simulink model "I_HeatConductionThroughInsulatedIronRod"  (R2024b)
settings: Solver=VariableStepAuto  StartTime=0.0  StopTime=5  MaxStep=100  RelTol=1e-3  AbsTol=1e-3  EnableMultiTasking=on
PreLoadFcn:
  | if ~exist('T_base', 'var')   T_base= 100;   end % [degC]
  | if ~exist('L', 'var')        L= 0.2;        end % [m]
  | if ~exist('D', 'var')        D= 0.025;      end % [m]
  | if ~exist('A', 'var')        A= pi*D^2/4;   end % [m^2]
  | if ~exist('k', 'var')        k= 80.2;       end % [W/(K*m)]
  | if ~exist('Q_case_1', 'var') Q_case_1= 18;  end % [W]
libraries: fl_lib x6, nesl_utility x2
Description:
  | Steady State Heat Conduction Through Insulated Iron Rod
settings Model: Creator=The MathWorks, Inc.  LastModifiedBy=mvahab
settings SolverCC: AutoScaleAbsTol=off  AlgebraicLoopSolver=TrustRegion
settings DataIOCC: LimitDataPoints=on  SaveFormat=Array  ReturnWorkspaceOutputs=off
settings OptimizationCC: LifeSpan=inf
settings DebuggingCC: SolverPrmCheckMsg=warning  UnconnectedInputMsg=warning  UnconnectedOutputMsg=warning  UnconnectedLineMsg=warning  AllowSymbolicDim=off  PregeneratedLibrarySubsystemCodeDiagnostic=none  SFUnexpectedBacktrackingDiag=warning  SFNoUnconditionalDefaultTransitionDiag=warning  SFExecutionAtInitializationDiag=none  ArithmeticOperatorsInVariantConditions=warning
settings HardwareCC: ProdBitPerPointer=32  ProdBitPerSizeT=32  ProdBitPerPtrDiffT=32  ProdLargestAtomicFloat=None  ProdIntDivRoundTo=Undefined  ProdEndianess=Unspecified  ProdWordSize=32  ProdHWDeviceType=32-bit Generic
settings ModelReferenceCC: EnableRefExpFcnMdlSchedulingChecks=on  PropagateSignalLabelsOutOfModel=off
settings SFSimCC: SimUseLocalCustomCode=off  CustomCodeUndefinedFunction=UseInterfaceOnly
settings RTWCC: RTWUseLocalCustomCode=off  GPUComputeCapability=3.5  DLArmComputeVersion=19.05
settings CodeAppCC: StateflowObjectComments=on
settings GRTTargetCC: TargetLangStandard=C89/C90 (ANSI)
settings ConfigComp: CovMetricSettings=dw  CovSaveCumulativeToWorkspaceVar=on  CovSaveSingleToWorkspaceVar=on  CovExternalEMLEnable=off  CovSFcnEnable=off
settings SimscapeCC: SimscapeLogType=all  SimscapeLogSimulationStatistics=on  SimscapeLogName=simlog_HeatConductionThroughInsulatedIronRod  SimscapeLogDataHistory=10000

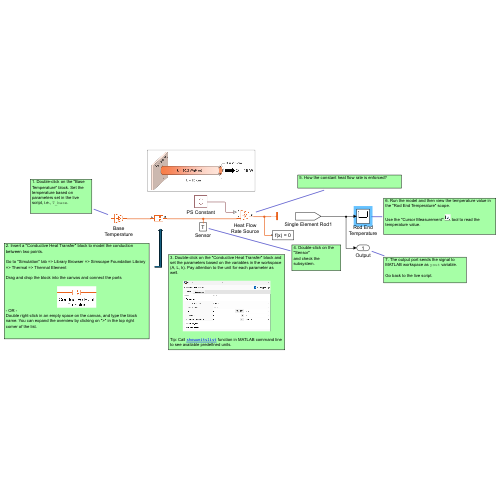
[thumbnail: Simulink's stored preview of the top-level diagram]
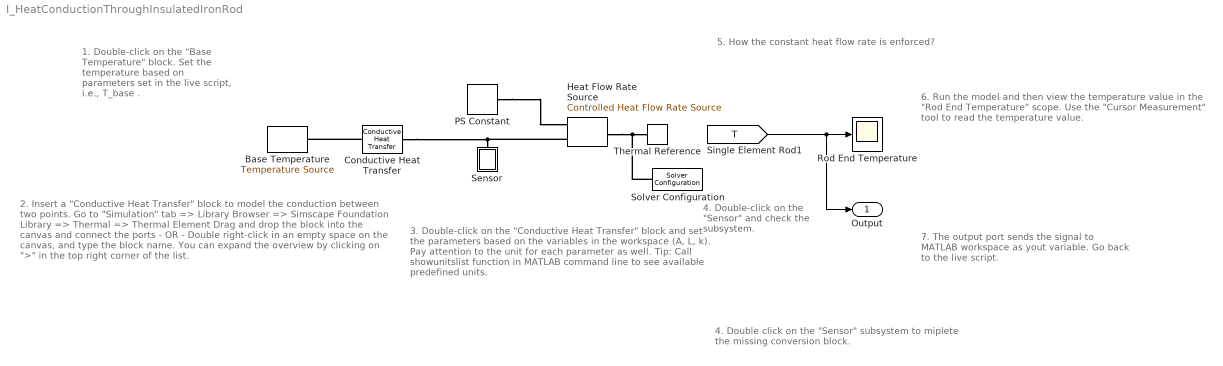
== system I_HeatConductionThroughInsulatedIronRod ==
  note: 2. Insert a "Conductive Heat Transfer" block to model the conduction between two points.
      |
      | Go to "Simulation" tab => Library Browser => Simscape Foundation Library => Thermal => Thermal Element
      |
      | Drag and drop the block into the canvas and connect the ports
      |
      | - OR -
      | Double right-click in an empty space on the canvas, and type the block name. You can expand the overview by clicking on ">" in the top right corner of the list.
  note: 3. Double-click on the "Conductive Heat Transfer" block and set the parameters based on the variables in the workspace (A, L, k). Pay attention to the unit for each parameter as well.
      |
      | Tip: Call showunitslist function in MATLAB command line to see available predefined units.
  note: 4. Double-click on the "Sensor"
      | and check the subsystem.
  note: 1. Double-click on the "Base Temperature" block. Set the temperature based on parameters set in the live script, i.e., T_base .
  note: 4. Double click on the "Sensor" subsystem to miplete the missing conversion block.
  note: 6. Run the model and then view the temperature value in the "Rod End Temperature" scope.
      |
      | Use the "Cursor Measurement" tool to read the temperature value.
  note: 7. The output port sends the signal to MATLAB workspace as yout variable.
      |
      | Go back to the live script.
  note: 5. How the constant heat flow rate is enforced?
  Base Temperature : fl_lib/Thermal/Thermal Sources/Temperature Source  temperature=T_base degC
  Conductive Heat Transfer : fl_lib/Thermal/Thermal Elements/Conductive Heat Transfer  thermal_type=foundation.enum.ConstantVariableTabulated.Constant  wall_geometry=foundation.enum.ConductionWallGeometry.Planar  area=A m^2  thickness=L m  d_in=0.05 m  d_out=0.1 m  L=1 m  th_cond_min=10 W/(K*m)  th_cond=k W/(K*m)  th_cond_TLU=[413, 401, 392, 383, 371, 357, 342] W/(K*m)  temp_TLU=[200, 273, 400, 600, 800, 1000, 1200] K  T_specify=off  T_priority=None  T=0 K  T_nominal_specify=off  T_nominal_value=1  T_nominal_unit=K  Q_specify=off  Q_priority=None  Q=0 W  Q_nominal_specify=off  Q_nominal_value=1  Q_nominal_unit=W
  Heat Flow Rate Source : fl_lib/Thermal/Thermal Sources/Controlled Heat Flow Rate Source
  PS Constant : fl_lib/Physical Signals/Sources/PS Constant  constant=Q_case_1 W
  Rod End Temperature : Scope
  Sensor : Subsystem
      mask Display: disp('T')
  Solver Configuration : nesl_utility/Solver Configuration  PhysicalDomain=network_engine_domain  SubClassName=solver  LeftPortType=input  RightPortType=generic  Tones=[]  Harmonics=[]  SimulateNoise=off  Profile=off  UseLocalSampling=off  EnableSwitchedLinearOptims=on  FrequencyDomain=off  UseCCode=off  RelTol=0.001  AbsTol=1e-06  MinStep=1e-09  ToWorkspace=off  RevertToSquareIcSolve=off  NumHomotopyIterations=100  PhasorMode=off  PhasorModeNumHarmonics=1  ConsistencySolver=NEWTON_XTOL_AFTER_FTOL  IndexReductionMethod=DerivativeReplacement  DoDC=off  ResidualTolerance=1e-9  ConsistencyTolSource=GLOBAL  ConsistencyAbsTol=0.001  ConsistencyRelTol=0.001  ConsistencyTolFactor=0.001  UseLocalSolver=off  LocalSolverChoice=NE_BACKWARD_EULER_ADVANCER  ResolveIndetEquations=on  FunctionEvalNumThread=1  LocalSolverSampleTime=.001  DoFixedCost=off  MaxNonlinIter=3  MaxModeIter=2  ComputeImpulses=off  ImpulseIterations=2  LinearAlgebra=auto  LinearAlgebraNumThread=0  EquationFormulation=NE_TIME_EF  DelaysMemoryBudget=1024  AutomaticFiltering=on  FilteringTimeConstant=0.001  PartitionStorageMethod=AS_NEEDED  PartitionMemoryBudget=1024  PartitionMethod=FAST  MultibodyUseLocalSolver=off  MultibodyLocalSolverChoice=ODE1  MultibodyLocalSolverSampleTime=0.001
  Thermal Reference : fl_lib/Thermal/Thermal Elements/Thermal Reference
  Output : Outport
  wires:
  [T] -> Output/1, Rod End Temperature/1
  connections:
  Conductive Heat Transfer/LConn1 -- Base Temperature/LConn1
  Heat Flow Rate Source/RConn2 -- Conductive Heat Transfer/RConn1 -- Sensor/LConn1
  Heat Flow Rate Source/LConn1 -- Solver Configuration/RConn1 -- Thermal Reference/LConn1
  PS Constant/RConn1 -- Heat Flow Rate Source/RConn1

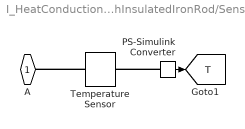
== system I_HeatConductionThroughInsulatedIronRod/Sensor ==
  PS-Simulink Converter : nesl_utility/PS-Simulink Converter  PhysicalDomain=network_engine_domain  SubClassName=ps_output  LeftPortType=input  RightPortType=output  PseudoPeriodic=off  Frequencies=[]  VectorFormat=1-D array  Unit=degC  AffineConversion=on
  Temperature Sensor : fl_lib/Thermal/Thermal Sensors/Temperature Sensor  temperature_measure=foundation.enum.MeasurementReference.absolute
      settings: InternalSimscapePortConfiguration="{\"Bottom\":[],\"Left\":[{\"id\":\"A\",\"label\":\"A\",\"type\":\"foundation.thermal.thermal\"}],\"Right\":[{\"id\":\"T\",\"label\":\"T\",\"type\":\"output\"}],\"Top\":[]}"
  A : PMIOPort  Side=Left
  tag scope: T=global
  wires:
  PS-Simulink Converter/1 -> [T]
  connections:
  PS-Simulink Converter/LConn1 -- Temperature Sensor/RConn1
  Temperature Sensor/LConn1 -- A/RConn1
